simulink model "model_1expV"  (R2023a)
settings: Solver=VariableStepAuto  StartTime=0.0  StopTime=150  RelTol=1e-3
values from neighbouring files (symbols this model uses):
  a = A(3)    [F1Vexp2V.m]    (also in F1Vexp2V_SexpS.m; F1Vexp2V_SexpS_ssr_all.m = input_parameters(3); F1Vexp3V.m; F1VexpV.m)
  data = load(input_data)    [F1.m]    (also in F1Sy.m; F1Vexp2V.m; F1Vexp2V_SexpS.m; F1Vexp2V_SexpS_ssr.m)
  R = A(2)    [F1.m]    (also in F1Sy.m; F1Vexp2V.m; F1Vexp2V_SexpS.m; F1Vexp2V_SexpS_ssr_all.m = input_parameters(2))
  x = input_parameters(1)    [F1Vexp2V_SexpS_ssr.m]    (also in F1Vexp2V_SexpS_ssr_all.m = input_parameters(4); F1Vexp2V_ssr.m; F1Vexp3V_ssr.m; F1VexpV_ssr.m)
settings Model: Creator=test  LastModifiedBy=test

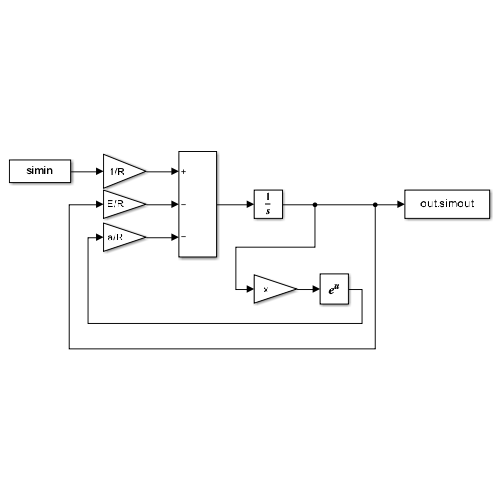
[thumbnail: Simulink's stored preview of the top-level diagram]
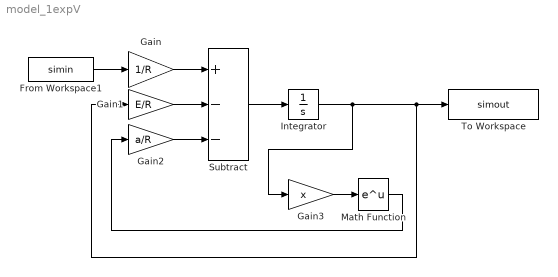
== system model_1expV ==
  From Workspace1 : FromWorkspace  VariableName=simin
  Gain : Gain  Gain=1/R
  Gain1 : Gain  Gain=E/R
  Gain2 : Gain  Gain=a/R
  Gain3 : Gain  Gain=x
  Integrator : Integrator  InitialCondition=data(1,3)
  Math Function : Math
  Subtract : Sum  Inputs=+--
  To Workspace : ToWorkspace  VariableName=simout  SaveFormat=Timeseries  SampleTime=0.01
  wires:
  Gain2/1 -> Subtract/3
  Gain/1 -> Subtract/1
  From Workspace1/1 -> Gain/1
  Math Function/1 -> Gain2/1
  Gain1/1 -> Subtract/2
  Subtract/1 -> Integrator/1
  Integrator/1 -> Gain3/1, Gain1/1, To Workspace/1
  Gain3/1 -> Math Function/1
